simulink model "Path_following_Model_w_dbl_lane_change"  (R2023a)
settings: Solver=VariableStepAuto  StartTime=0.0  StopTime=25  FixedStep=1  RelTol=1e-3
undefined symbols (not defined in the file): A_matrix, B_matrix, C_matrix, Cum_dis, D, D_matrix, dis_vec, I, N, P, path_curvatures, sigbuilder_block, V, Xp, Yp
libraries: simulink x1, slpidlib x1
settings Model: Creator=Santo  LastModifiedBy=brianlesko
settings SolverCC: AlgebraicLoopSolver=TrustRegion
settings DataIOCC: ReturnWorkspaceOutputs=off
settings OptimizationCC: ReuseModelBlockBuffer=off
settings DebuggingCC: UnconnectedInputMsg=warning  UnconnectedOutputMsg=warning  UnconnectedLineMsg=warning  ArithmeticOperatorsInVariantConditions=warning
settings ModelReferenceCC: EnableRefExpFcnMdlSchedulingChecks=on
settings SFSimCC: SimUseLocalCustomCode=off  CustomCodeUndefinedFunction=UseInterfaceOnly
settings RTWCC: RTWUseLocalCustomCode=off

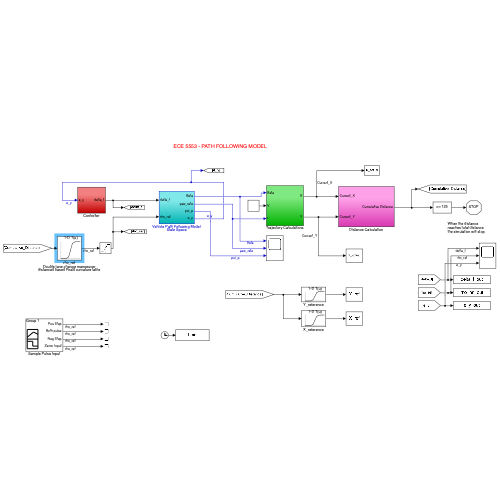
[thumbnail: Simulink's stored preview of the top-level diagram]
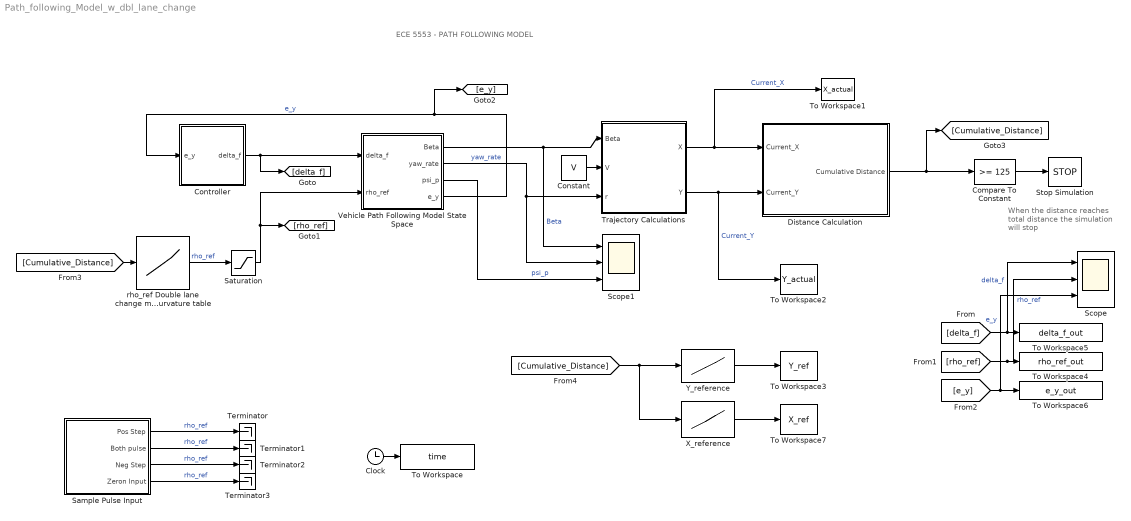
== system Path_following_Model_w_dbl_lane_change ==
  note: When the distance reaches total distance the simulation will stop
  note: ECE 5553 - PATH FOLLOWING MODEL
  Clock : Clock
  Compare To Constant : simulink/Logic and Bit Operations/Compare To Constant  relop=>=  const=125  OutDataTypeStr=boolean
  Constant : Constant  Value=V
  Controller : Subsystem
  Distance Calculation : Subsystem
  Sample Pulse Input : Subsystem  Tag=STV Subsys  LoadFcn=sigbuilder_block('load');  StartFcn=sigbuilder_block('start');  StopFcn=sigbuilder_block('stop');  ClipboardFcn=sigbuilder_block('clipboard');  mask(Sigbuilder block){tuvar=[0:10]}
      mask help: Simulink:masks:SigbuilderBlock_MD
      mask init:
      | if ~strcmp(get_param(bdroot(gcbh),'SimulationStatus'),'stopped') tuvar = sigbuilder_block('maskInit'); end
      settings: CopyFcn=sigbuilder_block('copy');  DeleteFcn=sigbuilder_block('delete');  ModelCloseFcn=sigbuilder_block('modelClose');  PreSaveFcn=sigbuilder_block('preSave');  PauseFcn=sigbuilder_block('pause');  ContinueFcn=sigbuilder_block('continue');  NameChangeFcn=sigbuilder_block('namechange');  OpenFcn=sigbuilder_block('open',[177 285 1013 454 ]);  CloseFcn=sigbuilder_block('close');
      mask Display: plot(0, 0, 100, 100,[2, 2, 32, 32, 2], [68, 8, 8, 68, 68],[32, 2], [38, 38], [32, 19, 2],[53, 60, 44], [32, 17, 17, 2],[16, 16, 31, 31]);txt = getActiveGroup(gcbh);text(2, 100, txt,'verticalAlignment', 'top');
  Saturation : Saturate  UpperLimit=0.01  LowerLimit=-0.025  LinearizeAsGain=off
  Scope : Scope  NumInputPorts=3
  Scope1 : Scope  NumInputPorts=3
  Stop Simulation : Stop
  Terminator{,1..3} (4 alike) : Terminator
  To Workspace : ToWorkspace  VariableName=time  SampleTime=-1
  To Workspace1 : ToWorkspace  VariableName=X_actual  SampleTime=-1
  To Workspace2 : ToWorkspace  VariableName=Y_actual  SampleTime=-1
  To Workspace3 : ToWorkspace  VariableName=Y_ref  SampleTime=-1
  To Workspace4 : ToWorkspace  VariableName=rho_ref_out  SampleTime=-1
  To Workspace5 : ToWorkspace  VariableName=delta_f_out  SampleTime=-1
  To Workspace6 : ToWorkspace  VariableName=e_y_out  SampleTime=-1
  To Workspace7 : ToWorkspace  VariableName=X_ref  SampleTime=-1
  Trajectory Calculations : Subsystem
  Vehicle Path Following Model State Space : Subsystem
  X_reference : Lookup_n-D  NumberOfTableDimensions=1  BreakpointsForDimension1=Cum_dis  Table=Xp(1:end-1)  InternalRulePriority=Speed  RndMeth=Simplest
  Y_reference : Lookup_n-D  NumberOfTableDimensions=1  BreakpointsForDimension1=Cum_dis  Table=Yp(1:end-1)  InternalRulePriority=Speed  RndMeth=Simplest
  rho_ref Double lane change manoeuver distanced based Road curvature table : Lookup_n-D  NumberOfTableDimensions=1  BreakpointsForDimension1=dis_vec  Table=path_curvatures  InternalRulePriority=Speed  RndMeth=Simplest
  wires:
  Trajectory Calculations/1(X) -> Distance Calculation/1(Current_X), To Workspace1/1  "Current_X"
  Constant/1 -> Trajectory Calculations/2(V)
  Vehicle Path Following Model State Space/4(e_y) -> [e_y], Controller/1(e_y)  "e_y"
  Vehicle Path Following Model State Space/1(Beta) -> Scope1/1, Trajectory Calculations/1(Beta)  "Beta"
  Vehicle Path Following Model State Space/2(yaw_rate) -> Scope1/2, Trajectory Calculations/3(r)  "yaw_rate"
  Controller/1(delta_f) -> [delta_f], Vehicle Path Following Model State Space/1(delta_f)
  [delta_f] -> Scope/1, To Workspace5/1  "delta_f"
  [rho_ref] -> Scope/2, To Workspace4/1  "rho_ref"
  [e_y] -> Scope/3, To Workspace6/1  "e_y"
  Vehicle Path Following Model State Space/3(psi_p) -> Scope1/3  "psi_p"
  Trajectory Calculations/2(Y) -> To Workspace2/1, Distance Calculation/2("Current_Y ")  "Current_Y"
  rho_ref Double lane change manoeuver distanced based Road curvature table/1 -> Saturation/1  "rho_ref"
  Compare To Constant/1 -> Stop Simulation/1
  Saturation/1 -> Vehicle Path Following Model State Space/2(rho_ref), [rho_ref]
  Distance Calculation/1(Cumulative Distance) -> [Cumulative_Distance], Compare To Constant/1
  Sample Pulse Input/1(Pos Step) -> Terminator/1  "rho_ref"
  Sample Pulse Input/2(Both pulse) -> Terminator1/1  "rho_ref"
  Sample Pulse Input/3(Neg Step) -> Terminator2/1  "rho_ref"
  Sample Pulse Input/4(Zeron Input) -> Terminator3/1  "rho_ref"
  X_reference/1 -> To Workspace7/1
  Y_reference/1 -> To Workspace3/1
  [Cumulative_Distance] -> rho_ref Double lane change manoeuver distanced based Road curvature table/1
  [Cumulative_Distance] -> X_reference/1, Y_reference/1
  Clock/1 -> To Workspace/1

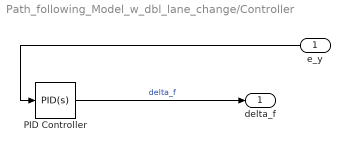
== system Path_following_Model_w_dbl_lane_change/Controller ==
  e_y : Inport
  PID Controller : slpidlib/PID Controller  Controller=PID  Form=Parallel  TimeDomain=Continuous-time  UseExternalTs=off  SampleTime=-1  IntegratorMethod=Forward Euler  FilterMethod=Forward Euler  ControllerParametersSource=internal  P=P  I=I  UseKiTs=off  D=D  N=N  UseFilter=on  TunerSelectOption=Transfer Function Based (PID Tuner App)  InitialConditionSource=internal  InitialConditionForIntegrator=0  InitialConditionForFilter=0  DifferentiatorICPrevScaledInput=0  ExternalReset=none  TrackingMode=off  Kt=1  LimitOutput=off  SatLimitsSource=internal  UpperSaturationLimit=inf  LowerSaturationLimit=-inf  LinearizeAsGain=on  AntiWindupMode=none  Kb=1  LimitIntegrator=off  UpperIntegratorSaturationLimit=inf  LowerIntegratorSaturationLimit=-inf  POutMin=[]  POutMax=[]  IOutMin=[]  IOutMax=[]  DOutMin=[]  DOutMax=[]  NOutMin=[]  NOutMax=[]  SumOutMin=[]  SumOutMax=[]  SaturationOutMin=[]  SaturationOutMax=[]  PParamMin=[]  PParamMax=[]  IParamMin=[]  IParamMax=[]  DParamMin=[]  DParamMax=[]  NParamMin=[]  NParamMax=[]  KbParamMin=[]  KbParamMax=[]  KtParamMin=[]  KtParamMax=[]  KbOutMin=[]  KbOutMax=[]  KtOutMin=[]  KtOutMax=[]  IntegratorOutMin=[]  IntegratorOutMax=[]  FilterOutMin=[]  FilterOutMax=[]  SumI1OutMin=[]  SumI1OutMax=[]  SumI2OutMin=[]  SumI2OutMax=[]  SumI3OutMin=[]  SumI3OutMax=[]  SumI4OutMin=[]  SumI4OutMax=[]  SumDOutMin=[]  SumDOutMax=[]  DifferentiatorOutMin=[]  DifferentiatorOutMax=[]  FilterDiffOutCoefMin=[]  FilterDiffOutCoefMax=[]  ReciprocalOutMin=[]  ReciprocalOutMax=[]  SumDenOutMin=[]  SumDenOutMax=[]  SumNumOutMin=[]  SumNumOutMax=[]  DivideOutMin=[]  DivideOutMax=[]  UdiffTsProdOutMin=[]  UdiffTsProdOutMax=[]  NTsProdOutMin=[]  NTsProdOutMax=[]  UintegralTsProdOutMin=[]  UintegralTsProdOutMax=[]  UngainTsProdOutMin=[]  UngainTsProdOutMax=[]  ClampingZeroOutDataTypeStr=Inherit: Inherit via back propagation  ClampingZeroOutMin=[]  ClampingZeroOutMax=[]  FilterDenConstantOutDataTypeStr=Inherit: Inherit via back propagation  FilterDenConstantOutMin=[]  FilterDenConstantOutMax=[]  PCopyOutDataTypeStr=Inherit: Inherit via back propagation  PCopyOutMin=[]  PCopyOutMax=[]  NCopyOutDataTypeStr=Inherit: Inherit via back propagation  NCopyOutMin=[]  NCopyOutMax=[]  IntegratorContinuousStateAttributes=''  IntegratorStateMustResolveToSignalObject=off  IntegratorRTWStateStorageClass=Auto  FilterContinuousStateAttributes=''  FilterStateMustResolveToSignalObject=off  FilterRTWStateStorageClass=Auto  ParallelPVariant=InternalParameters  IdealPVariant=Disabled  IVariant=InternalParameters  DVariant=InternalParameters  IntegratorVariant=Continuous  SatVariant=Disabled  AWVariant=Passthrough  PCopyVariant=Disabled  TRVariant=Disabled  FdbkBlocksVariant=Forward  IdealPFdbkVariant=Disabled  SatFdbkVariant=Disabled  DerivativeFilterVariant=ContFilter  NVariant=InternalParameters  NCopyVariant=Disabled  FilterICVariant=InternalICsFilter  IntegratorICVariant=InternalICs  ExternalResetVariant=Disabled  TRSumVariant=Passthrough  SumFdbkVariant=Disabled  SumVariant=Sum_PID  TsampFilterVariant=InternalTs  TsampNgainVariant=Passthrough  TsampIntegralVariant=Disabled_SignalSpec  ExternalSaturationOutDataTypeStr=Inherit: Same as second input
  delta_f : Outport  VectorParamsAs1DForOutWhenUnconnected=off
  wires:
  PID Controller/1 -> delta_f/1  "delta_f"
  e_y/1 -> PID Controller/1

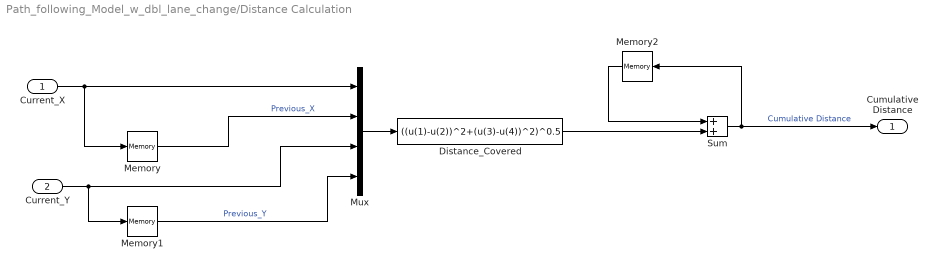
== system Path_following_Model_w_dbl_lane_change/Distance Calculation ==
  Current_X : Inport
  "Current_Y " : Inport  Port=2
  Distance_Covered : Fcn  Expr=((u(1)-u(2))^2+(u(3)-u(4))^2)^0.5
  Memory : Memory
  Memory1 : Memory
  Memory2 : Memory
  Mux : Mux
  Sum : Sum
  Cumulative Distance : Outport  VectorParamsAs1DForOutWhenUnconnected=off
  wires:
  Memory1/1 -> Mux/4  "Previous_Y"
  Mux/1 -> Distance_Covered/1
  Distance_Covered/1 -> Sum/2
  Memory/1 -> Mux/2  "Previous_X"
  Memory2/1 -> Sum/1
  "Current_Y "/1 -> Memory1/1, Mux/3
  Current_X/1 -> Memory/1, Mux/1
  Sum/1 -> Cumulative Distance/1, Memory2/1  "Cumulative Distance"

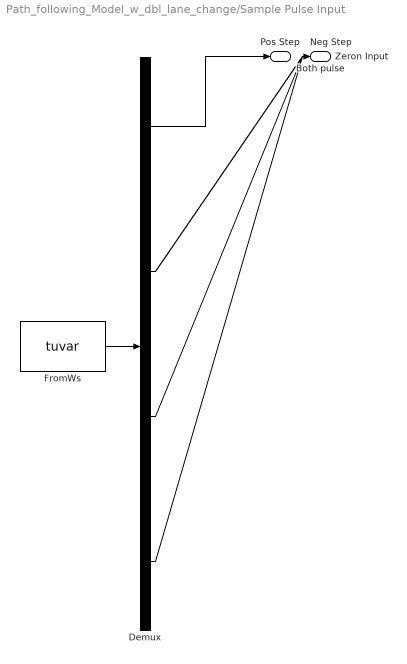
== system Path_following_Model_w_dbl_lane_change/Sample Pulse Input ==
  Demux : Demux  Tag=STV Demux
      settings: DisplayOption=none
  FromWs : FromWorkspace  Tag=STV FromWs  VariableName=tuvar
      SigBuilderData=|
      | common.afterFinalStr = 'Extrapolate'
      | common.sampleTime = 0
      | dataSet.timeRange = [0 10]
      | dataSet.name = 'Group 1'
      | sbobj.Groups.Name = 'Group 1'
      | sbobj.Groups.Signals(1).Name = 'Pos Step'
      | sbobj.Groups.Signals(1).XData = [0 4 4 6 6 10]
      | sbobj.Groups.Signals(1).YData = [0 0 0.1 0.1 0 0]
      | sbobj.Groups.Signals(2).Name = 'Both pulse'
      | sbobj.Groups.Signals(2).XData = [0 4 4 6 6 7 7 9 9 10]
      | sbobj.Groups.Signals(2).YData = [0 0 0.1 0.1 0 0 -0.1 -0.1 0 0]
      | sbobj.Groups.Signals(3).Name = 'Neg Step'
      | sbobj.Groups.Signals(3).XData = [0 4 4 6 6 10]
      | sbobj.Groups.Signals(3).YData = [0 0 -0.1 -0.1 0 0]
      | sbobj.Groups.Signals(4).Name = 'Zeron Input'
      | sbobj.Groups.Signals(4).XData = [0 10]
      | sbobj.Groups.Signals(4).YData = [0 0]
  Pos Step : Outport  Tag=STV Outport  VectorParamsAs1DForOutWhenUnconnected=off
  Both pulse : Outport  Tag=STV Outport  Port=2  VectorParamsAs1DForOutWhenUnconnected=off
  Neg Step : Outport  Tag=STV Outport  Port=3  VectorParamsAs1DForOutWhenUnconnected=off
  Zeron Input : Outport  Tag=STV Outport  Port=4  VectorParamsAs1DForOutWhenUnconnected=off
  wires:
  FromWs/1 -> Demux/1
  Demux/1 -> Pos Step/1
  Demux/2 -> Both pulse/1
  Demux/3 -> Neg Step/1
  Demux/4 -> Zeron Input/1

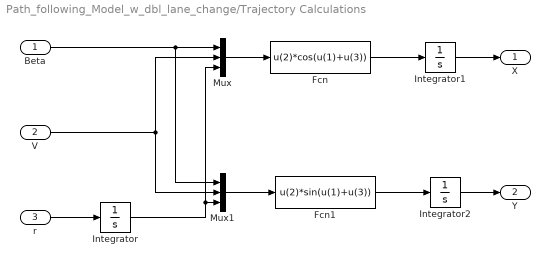
== system Path_following_Model_w_dbl_lane_change/Trajectory Calculations ==
  Beta : Inport
  V : Inport  Port=2
  r : Inport  Port=3
  Fcn : Fcn  Expr=u(2)*cos(u(1)+u(3))
  Fcn1 : Fcn  Expr=u(2)*sin(u(1)+u(3))
  Integrator : Integrator
  Integrator1 : Integrator  InitialCondition=Xp(1)
  Integrator2 : Integrator  InitialCondition=Yp(1)
  Mux : Mux  Inputs=3
  Mux1 : Mux  Inputs=3
  X : Outport  VectorParamsAs1DForOutWhenUnconnected=off
  Y : Outport  Port=2  VectorParamsAs1DForOutWhenUnconnected=off
  wires:
  Integrator2/1 -> Y/1
  Fcn1/1 -> Integrator2/1
  Integrator1/1 -> X/1
  Fcn/1 -> Integrator1/1
  Mux1/1 -> Fcn1/1
  Mux/1 -> Fcn/1
  Integrator/1 -> Mux1/3, Mux/3
  V/1 -> Mux1/2, Mux/2
  Beta/1 -> Mux1/1, Mux/1
  r/1 -> Integrator/1

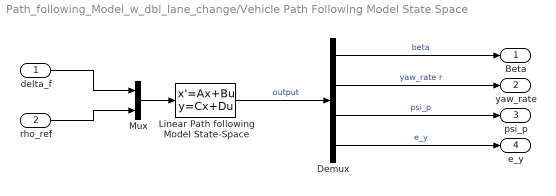
== system Path_following_Model_w_dbl_lane_change/Vehicle Path Following Model State Space ==
  delta_f : Inport
  rho_ref : Inport  Port=2
  Demux : Demux
  Linear Path following Model State-Space : StateSpace  A=A_matrix  B=B_matrix  C=C_matrix  D=D_matrix  InitialCondition=0
  Mux : Mux  Inputs=2
  Beta : Outport  VectorParamsAs1DForOutWhenUnconnected=off
  yaw_rate : Outport  Port=2  VectorParamsAs1DForOutWhenUnconnected=off
  psi_p : Outport  Port=3  VectorParamsAs1DForOutWhenUnconnected=off
  e_y : Outport  Port=4  VectorParamsAs1DForOutWhenUnconnected=off
  wires:
  Demux/4 -> e_y/1  "e_y"
  Mux/1 -> Linear Path following Model State-Space/1
  Demux/2 -> yaw_rate/1  "yaw_rate r"
  Linear Path following Model State-Space/1 -> Demux/1  "output"
  Demux/1 -> Beta/1  "beta"
  rho_ref/1 -> Mux/2
  delta_f/1 -> Mux/1
  Demux/3 -> psi_p/1  "psi_p"
